simulink model "TASK8_3"  (R2019a)
settings: Solver=VariableStepAuto  StartTime=0.0  StopTime=30  RelTol=1e-3
values from neighbouring files (symbols this model uses):
  Ct = [0 0 0 1]    [Dharmesh_DCS_LAB_Script.m]
  g = 9.81    [Dharmesh_DCS_LAB_Script.m]
  h = 0.1    [Dharmesh_DCS_LAB_Script.m]
  Jconst = Jb+mf*h^2    (= 0.501)    [Dharmesh_DCS_LAB_Script.m]
  Ki = Kpi(1:4)-(P*Ct)    [Dharmesh_DCS_LAB_Script.m]
  Kt_o_new = Kt_o.'    [Dharmesh_DCS_LAB_Script.m]
  mf = 0.1    [Dharmesh_DCS_LAB_Script.m]
  P = 1/(Ct*inv((B*K)-A)*B)    [Dharmesh_DCS_LAB_Script.m]
  Pi = -Kpi(5)    [Dharmesh_DCS_LAB_Script.m]
  Ts = 125e-6    (= 0.000125)    [Dharmesh_DCS_LAB_Script.m]
undefined symbols (not defined in the file or in its folder): AD, BD
settings Model: Creator=Admin  LastModifiedBy=Admin

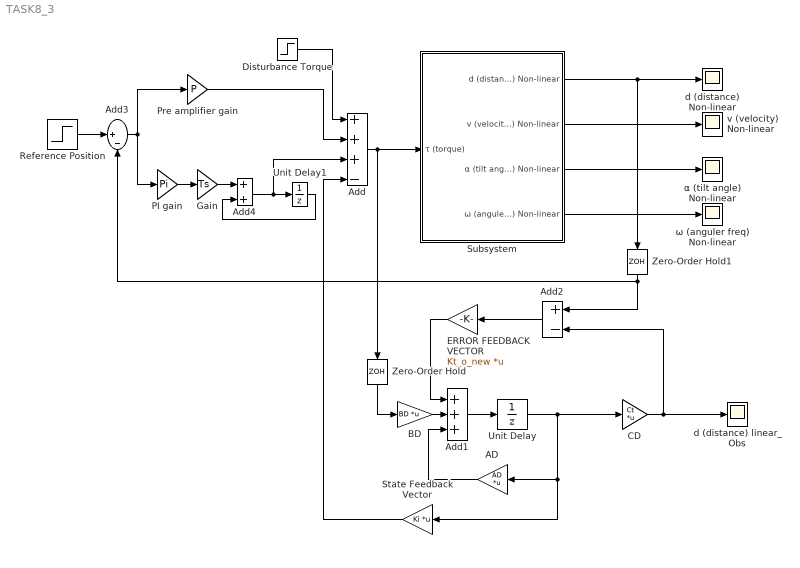
== system TASK8_3 ==
  AD : Gain  Gain=AD  Multiplication=Matrix(K*u) (u vector)
  Add : Sum  Inputs=+++-
  Add1 : Sum  Inputs=+++
  Add2 : Sum  Inputs=+-
  Add3 : Sum  Inputs=|+-
  Add4 : Sum
  BD : Gain  Gain=BD  Multiplication=Matrix(K*u) (u vector)
  CD : Gain  Gain=Ct  Multiplication=Matrix(K*u) (u vector)
  Disturbance Torque : Step  Time=15  After=0.1  SampleTime=0
  ERROR FEEDBACK VECTOR : Gain  Gain=Kt_o_new  Multiplication=Matrix(K*u) (u vector)
  Gain : Gain  Gain=Ts
  PI gain : Gain  Gain=Pi
  Pre amplifier gain : Gain  Gain=P
  Reference Position : Step  Time=0  SampleTime=0
  State Feedback Vector : Gain  Gain=Ki  Multiplication=Matrix(K*u) (u vector)
  Subsystem : Subsystem
  Unit Delay : UnitDelay  InitialCondition=[0;0;0;0.1]  SampleTime=Ts  HasFrameUpgradeWarning=on
  Unit Delay1 : UnitDelay  SampleTime=Ts  HasFrameUpgradeWarning=on
  Zero-Order Hold : ZeroOrderHold  SampleTime=Ts
  Zero-Order Hold1 : ZeroOrderHold  SampleTime=Ts
  d (distance) Non-linear : Scope
  d (distance) linear_Obs : Scope
  v (velocity) Non-linear : Scope
  α (tilt angle) Non-linear : Scope
  ω (anguler freq) Non-linear : Scope
  wires:
  Add1/1 -> Unit Delay/1
  PI gain/1 -> Gain/1
  Disturbance Torque/1 -> Add/1
  Unit Delay1/1 -> Add4/2
  Add3/1 -> PI gain/1, Pre amplifier gain/1
  State Feedback Vector/1 -> Add/4
  Zero-Order Hold1/1 -> Add3/2, Add2/1
  Zero-Order Hold/1 -> BD/1
  AD/1 -> Add1/3
  BD/1 -> Add1/2
  Add/1 -> Subsystem/1(τ (torque)), Zero-Order Hold/1
  Gain/1 -> Add4/1
  Reference Position/1 -> Add3/1
  Add2/1 -> ERROR FEEDBACK VECTOR/1
  ERROR FEEDBACK VECTOR/1 -> Add1/1
  Subsystem/1(d (distance) Non-linear) -> Zero-Order Hold1/1, d (distance) Non-linear/1
  Add4/1 -> Add/3, Unit Delay1/1
  Pre amplifier gain/1 -> Add/2
  CD/1 -> Add2/2, d (distance) linear_Obs/1
  Subsystem/2(v (velocity) Non-linear) -> v (velocity) Non-linear/1
  Subsystem/4(ω (anguler freq) Non-linear) -> ω (anguler freq) Non-linear/1
  Subsystem/3(α (tilt angle) Non-linear) -> α (tilt angle) Non-linear/1
  Unit Delay/1 -> State Feedback Vector/1, AD/1, CD/1

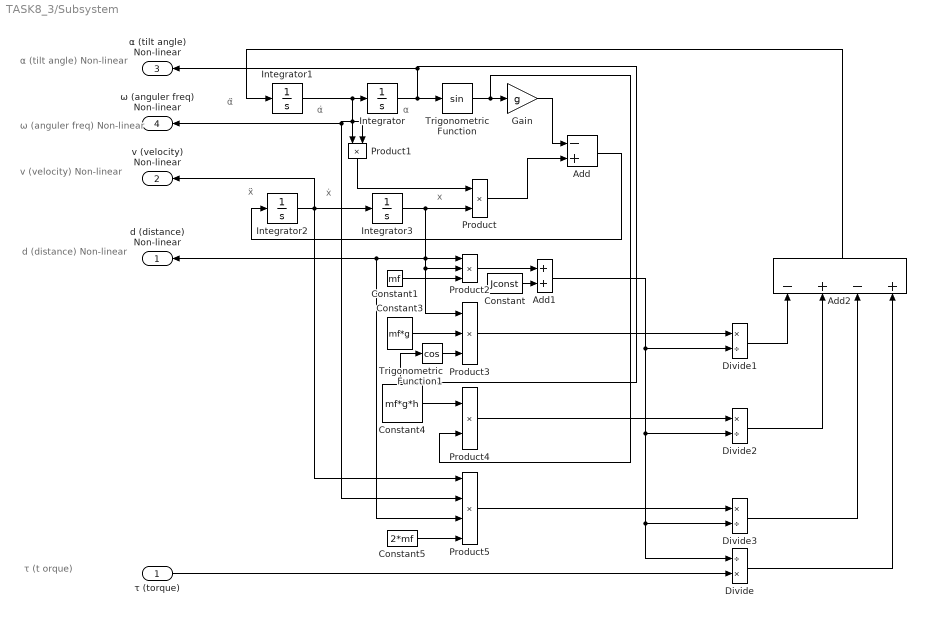
== system TASK8_3/Subsystem ==
  note: α̇
  note: α
  note: ẍ
  note: ẋ
  note: x
  note: τ (t orque)
  note: d (distance) Non-linear
  note: v (velocity) Non-linear
  note: α (tilt angle) Non-linear
  note: ω (anguler freq) Non-linear
  note: α̈
  τ (torque) : Inport
  Add : Sum  Inputs=-+
  Add1 : Sum
  Add2 : Sum  Inputs=-+-+
  Constant : Constant  Value=Jconst
  Constant1 : Constant  Value=mf
  Constant3 : Constant  Value=mf*g
  Constant4 : Constant  Value=mf*g*h
  Constant5 : Constant  Value=2*mf
  Divide : Product  Inputs=/*
  Divide1 : Product  Inputs=*/
  Divide2 : Product  Inputs=*/
  Divide3 : Product  Inputs=*/
  Gain : Gain  Gain=g
  Integrator{,1..3} (4 alike) : Integrator
  Product : Product
  Product1 : Product
  Product2 : Product  Inputs=3
  Product3 : Product  Inputs=3
  Product4 : Product
  Product5 : Product  Inputs=4
  Trigonometric Function : Trigonometry
  Trigonometric Function1 : Trigonometry  Operator=cos
  d (distance) Non-linear : Outport
  v (velocity) Non-linear : Outport  Port=2
  α (tilt angle) Non-linear : Outport  Port=3
  ω (anguler freq) Non-linear : Outport  Port=4
  wires:
  Product2/1 -> Add1/1
  Integrator1/1 -> Product1/2, Product1/1, ω (anguler freq) Non-linear/1, Product5/2, Integrator/1
  Product5/1 -> Divide3/1
  Divide3/1 -> Add2/3
  Product4/1 -> Divide2/1
  Divide/1 -> Add2/4
  Integrator/1 -> Trigonometric Function1/1, α (tilt angle) Non-linear/1, Trigonometric Function/1
  Divide1/1 -> Add2/1
  Product1/1 -> Product/1
  Add1/1 -> Divide/1, Divide3/2, Divide2/2, Divide1/2
  Add/1 -> Integrator2/1
  Trigonometric Function/1 -> Product4/2, Gain/1
  Constant1/1 -> Product2/3
  Product3/1 -> Divide1/1
  Constant3/1 -> Product3/2
  Add2/1 -> Integrator1/1
  Integrator3/1 -> Product/2, Product3/1, Product2/2, d (distance) Non-linear/1, Product5/3, Product2/1
  Divide2/1 -> Add2/2
  Constant4/1 -> Product4/1
  Integrator2/1 -> v (velocity) Non-linear/1, Product5/1, Integrator3/1
  Constant/1 -> Add1/2
  Product/1 -> Add/2
  τ (torque)/1 -> Divide/2
  Constant5/1 -> Product5/4
  Trigonometric Function1/1 -> Product3/3
  Gain/1 -> Add/1
